simulink model "Block_Osl"  (R2022a)
settings: Solver=ode23tb  StartTime=0.0  StopTime=5  MaxStep=1e-4  RelTol=1e-5
libraries: dspswit3 x1, simulink x1
settings Model: Creator=админ  LastModifiedBy=админ

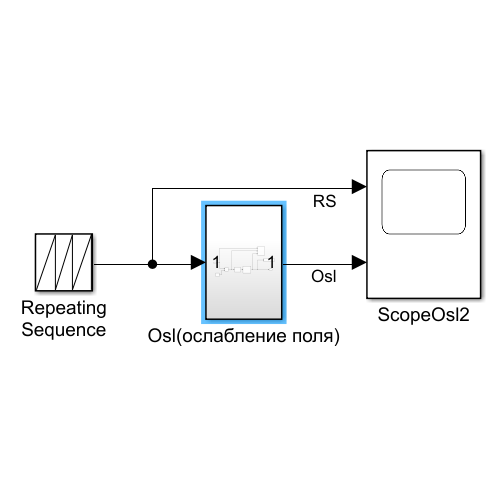
[thumbnail: Simulink's stored preview of the top-level diagram]
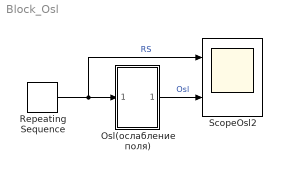
== system Block_Osl ==
  Osl(ослабление поля) : Subsystem
  Repeating Sequence : simulink/Sources/Repeating Sequence  rep_seq_t=Osl.RepSec.Time  rep_seq_y=Osl.RepSec.Output
  ScopeOsl2 : Scope  NumInputPorts=2
  wires:
  Repeating Sequence/1 -> ScopeOsl2/1, Osl(ослабление поля)/1(In1)  "RS"
  Osl(ослабление поля)/1(Out1) -> ScopeOsl2/2  "Osl"

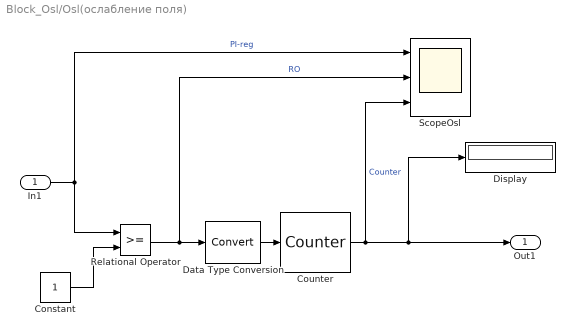
== system Block_Osl/Osl(ослабление поля) ==
  In1 : Inport
  Constant : Constant
  Counter : dspswit3/Counter  Direction=Up  CountEvent=Rising edge  CounterSize=User defined  MaxCount=Osl.Counter_MaxCount  InitialCount=0  Output=Count  HitValue=32  ResetInput=off  SamplesPerFrame=1  Ts=1  CntDtype=double  HitDtype=Logical
  Data Type Conversion : DataTypeConversion  SaturateOnIntegerOverflow=off  RndMeth=Floor
  Display : Display
  Relational Operator : RelationalOperator  OutDataTypeStr=boolean  RndMeth=Simplest  InputSameDT=off
  ScopeOsl : Scope  NumInputPorts=3
  Out1 : Outport
  wires:
  Counter/1 -> Out1/1, Display/1, ScopeOsl/3  "Counter"
  Relational Operator/1 -> ScopeOsl/2, Data Type Conversion/1  "RO"
  Constant/1 -> Relational Operator/2
  In1/1 -> Relational Operator/1, ScopeOsl/1  "PI-reg"
  Data Type Conversion/1 -> Counter/1
